simulink model "testfcn1"  (R2016b)
settings: Solver=VariableStepAuto  StartTime=0.0  StopTime=10.0  RelTol=1e-3
undefined symbols (not defined in the file or in its folder): VehState_MATLABStruct
settings Model: Creator=sgopalswamy  LastModifiedBy=sgopalswamy

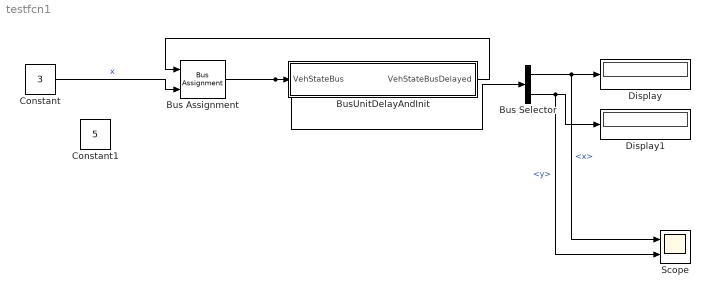
== system testfcn1 ==
  Bus Assignment : BusAssignment  AssignedSignals=x
  Bus Selector : BusSelector  OutputSignals=x,y
  BusUnitDelayAndInit : Subsystem
  Constant : Constant  Value=3
  Constant1 : Constant  Value=5
  Display : Display
  Display1 : Display
  Scope : Scope  NumInputPorts=2
  wires:
  Bus Selector/1 -> Scope/1, Display/1  "<x>"
  Bus Selector/2 -> Scope/2, Display1/1  "<y>"
  Constant/1 -> Bus Assignment/2  "x"
  Bus Assignment/1 -> Bus Selector/1, BusUnitDelayAndInit/1(VehStateBus)
  BusUnitDelayAndInit/1(VehStateBusDelayed) -> Bus Assignment/1

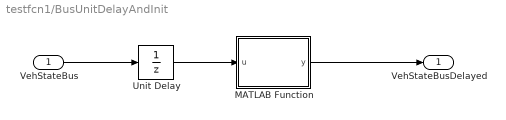
== system testfcn1/BusUnitDelayAndInit ==
  VehStateBus : Inport
  MATLAB Function : MATLAB Function  TreatAsAtomicUnit=on
  Unit Delay : UnitDelay  InitialCondition=VehState_MATLABStruct  SampleTime=-1
  VehStateBusDelayed : Outport
  wires:
  Unit Delay/1 -> MATLAB Function/1(u)
  VehStateBus/1 -> Unit Delay/1
  MATLAB Function/1(y) -> VehStateBusDelayed/1

== matlab function testfcn1/BusUnitDelayAndInit/MATLAB Function ==
  data: u input; y output Bus: VehState; VehState_MATLABStruct parameter
function y = testfcn1(u, VehState_MATLABStruct)
coder.extrinsic('exist')
persistent a
y0 = struct;
y0.x = 1;
y0.y = 2;
y0.z = 0;
y0.theta = 0;
y0.phi = 0;
y0.psi = 0;
y0.u = 0;
y0.v = 0;
y0.w = 0;
y0.dtheta = 0;
y0.dphi = 0;
y0.dpsi = 0;

%y0 = VehState_MATLABStruct;
if isempty(a)
    a = 1;
    y = y0;
else
    y = u;
end
